simulink model "Parkhaus_graphical_function"  (Simulink 4.00)
settings: Solver=FixedStepDiscrete  StartTime=0.0  StopTime=1000000000  FixedStep=0.01  RelTol=1e-3
libraries: simulink3 x2
settings Model: LastModifiedBy=Administrator  BlockReductionOpt=off

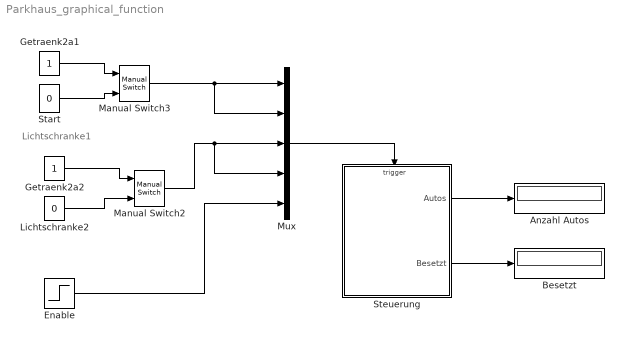
== system Parkhaus_graphical_function ==
  note: Lichtschranke1
  Anzahl Autos : Display
      settings: Format=short
  Besetzt : Display
      settings: Format=short
  Enable : Step  Time=1  Before=0  After=1  SampleTime=0
  Getraenk2a1 : Constant  Value=1
  Getraenk2a2 : Constant  Value=1
  Lichtschranke2 : Constant  Value=0
  Manual Switch2 : simulink3/Nonlinear/Manual Switch  sw=0  action=0
  Manual Switch3 : simulink3/Nonlinear/Manual Switch  sw=0  action=0
  Mux : Mux  Inputs=5
  Start : Constant  Value=0
  Steuerung : Stateflow chart  TreatAsAtomicUnit=on
      settings: RTWFcnNameOpts=Auto  RTWFileNameOpts=Auto
  wires:
  Mux/1 -> Steuerung/Trigger
  Lichtschranke2/1 -> Manual Switch2/2
  Getraenk2a2/1 -> Manual Switch2/1
  Start/1 -> Manual Switch3/2
  Manual Switch3/1 -> Mux/1, Mux/2
  Steuerung/1(Autos) -> Anzahl Autos/1
  Getraenk2a1/1 -> Manual Switch3/1
  Steuerung/2(Besetzt) -> Besetzt/1
  Manual Switch2/1 -> Mux/3, Mux/4
  Enable/1 -> Mux/5

== stateflow chart Steuerung ==
  state Idle
    entry:
    Besetzt=parkhaus2(Autos,Plaetze)
  state ZE1
  state ZA3
  state ZE2
  state ZE3
  state ZA1
  state ZA2
  state y = parkhaus2(a1,a2) [function]
    (default) -> (junction 11)
    (junction 11) -> (junction 13) : [a1<a2]{y=0;}
    (junction 11) -> (junction 12) : [a1>=a2]{y=1;}
  (default) -> Idle
  Idle -> ZE1 : a
  Idle -> ZA1 : c
  ZE1 -> ZE2 : c
  ZE1 -> Idle : b
  ZA1 -> Idle : d
  ZA1 -> ZA2 : a
  ZA2 -> ZA3 : d
  ZE3 -> Idle : d/Autos++
  ZE2 -> ZE1 : d
  ZA2 -> ZA1 : b
  ZA3 -> ZA2 : c
  ZE2 -> ZE3 : b
  ZE3 -> ZE2 : a
  ZA3 -> Idle : b/Autos--
  data: y function_output double; a1 function_input double; a2 function_input double; Autos output int16; Besetzt output int16; Plaetze constant int16 =5
  events: a input RISING_EDGE_EVENT; b input FALLING_EDGE_EVENT; c input RISING_EDGE_EVENT; d input FALLING_EDGE_EVENT; Enable input EITHER_EDGE_EVENT
